simulink model "modelado_pendulo"  (R2020a)
settings: Solver=ode15s  StartTime=0.0  StopTime=10.0  MaxStep=0.01  RelTol=1e-3
values from neighbouring files (symbols this model uses):
  b = 0.1    [fcn_transf_pend.m]    (also in modelado_pendulo_estados.m)
  g = 9.8    [fcn_transf_pend.m]    (also in modelado_pendulo_estados.m)
  I = 0.006    [fcn_transf_pend.m]    (also in modelado_pendulo_estados.m)
  l = 0.3    [fcn_transf_pend.m]    (also in modelado_pendulo_estados.m)
  m = 0.2    [fcn_transf_pend.m]    (also in modelado_pendulo_estados.m)
  M = 0.5    [fcn_transf_pend.m]    (also in modelado_pendulo_estados.m)
settings Model: Creator=rolan  LastModifiedBy=rolan

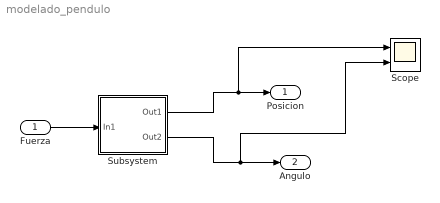
== system modelado_pendulo ==
  Fuerza : Inport
  Scope : Scope  NumInputPorts=2
  Subsystem : Subsystem
  Posicion : Outport
  Angulo : Outport  Port=2
  wires:
  Fuerza/1 -> Subsystem/1(In1)
  Subsystem/1(Out1) -> Scope/1, Posicion/1
  Subsystem/2(Out2) -> Scope/2, Angulo/1

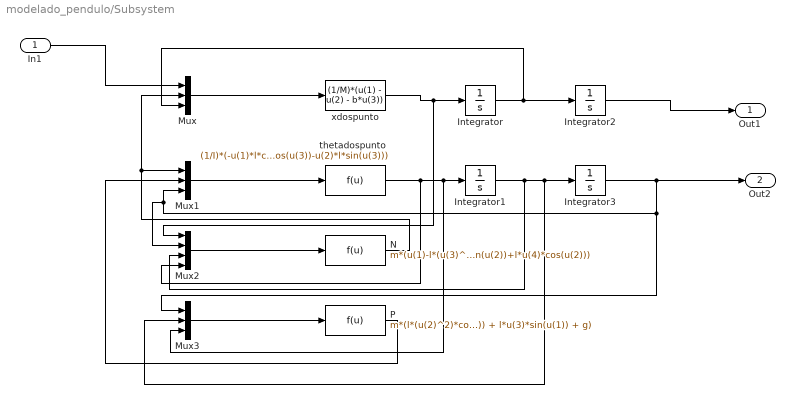
== system modelado_pendulo/Subsystem ==
  In1 : Inport
  Integrator : Integrator  ContinuousStateAttributes='xpunto'
  Integrator1 : Integrator  ContinuousStateAttributes='thetapunto'
  Integrator2 : Integrator  ContinuousStateAttributes='x'
  Integrator3 : Integrator  InitialCondition=pi  ContinuousStateAttributes='theta'
  Mux : Mux  Inputs=3
  Mux1 : Mux  Inputs=3
  Mux2 : Mux
  Mux3 : Mux  Inputs=3
  N : Fcn  Expr=m*(u(1)-l*(u(3)^2)*sin(u(2))+l*u(4)*cos(u(2)))
  P : Fcn  Expr=m*(l*(u(2)^2)*cos(u(1)) + l*u(3)*sin(u(1)) + g)
  thetadospunto : Fcn  Expr=(1/I)*(-u(1)*l*cos(u(3))-u(2)*l*sin(u(3)))
  xdospunto : Fcn  Expr=(1/M)*(u(1) - u(2) - b*u(3))
  Out1 : Outport
  Out2 : Outport  Port=2
  wires:
  Integrator3/1 -> Out2/1, Mux3/1, Mux2/2, Mux1/3
  Mux1/1 -> thetadospunto/1
  thetadospunto/1 -> Mux2/4, Mux3/3, Integrator1/1
  In1/1 -> Mux/1
  Integrator1/1 -> Mux2/3, Mux3/2, Integrator3/1
  Integrator/1 -> Mux/3, Integrator2/1
  P/1 -> Mux1/2
  N/1 -> Mux1/1, Mux/2
  xdospunto/1 -> Mux2/1, Integrator/1
  Mux3/1 -> P/1
  Mux/1 -> xdospunto/1
  Mux2/1 -> N/1
  Integrator2/1 -> Out1/1
